simulink model "ROCR6II_URDF_file_915"  (R2020b)
settings: Solver=VariableStepAuto  StartTime=0.0  StopTime=10  FixedStep=0.01  RelTol=1e-3
values from neighbouring files (symbols this model uses):
  X = [x,y,z,Roll,Pitch,Yaw]    [T2RPY.m]
undefined symbols (not defined in the file or in its folder): A, Y, Z
libraries: fl_lib x115, sm_lib x74, nesl_utility x59, fl_ps_legacy_lib x48, ee_lib x12, simulink_extras x7, simulink x6
(part 4 of 5)

== system ROCR6II_URDF_file_915/Driver1/Joint_Driver_5/Controller/Speed/Step Rate and Direction ==
  note: The speed controller turns the reference input into an absolute voltage demand for the
      | voltage-controlled pulse generator and sets the reverse flag signal to +5 volts when the
      | speed demand is negative.
  Reference : Inport
  Abs : Abs
  Compare To Constant : simulink/Logic and Bit Operations/Compare To Constant  relop=<  const=0  OutDataTypeStr=uint8  ZeroCross=off
  Data Type Conversion : DataTypeConversion
  IC Analog Output REV : Subsystem
  IC Analog Output Vref : Subsystem
  Logic2Volts : Gain  Gain=5
  Max step rate 100/s : Saturate  UpperLimit=100  LowerLimit=0
  StepRate2Volts : Gain  Gain=5/100
  REV : PMIOPort  Side=Right
  Vref : PMIOPort  Port=2  Side=Right
  wires:
  Logic2Volts/1 -> IC Analog Output REV/1(SL)
  Abs/1 -> Max step rate 100/s/1
  Reference/1 -> Abs/1, Compare To Constant/1
  Compare To Constant/1 -> Data Type Conversion/1
  Data Type Conversion/1 -> Logic2Volts/1
  Max step rate 100/s/1 -> StepRate2Volts/1
  StepRate2Volts/1 -> IC Analog Output Vref/1(SL)
  connections:
  Vref/RConn1 -- IC Analog Output Vref/RConn1
  REV/RConn1 -- IC Analog Output REV/RConn1

== system ROCR6II_URDF_file_915/Driver1/Joint_Driver_5/Controller/Speed/Voltage-Controlled Pulse Generator ==
  2*pi : fl_ps_legacy_lib/Legacy Physical Signals/Functions/PS Gain  gain=-2*pi
      settings: SourceProductName=Foundation Library
  Controlled Voltage Source : fl_lib/Electrical/Electrical Sources/Controlled Voltage Source
      settings: SourceProductName=Foundation Library
  ERef : fl_lib/Electrical/Electrical Elements/Electrical Reference
      settings: SourceProductName=Foundation Library
  Max step rate =100 : fl_ps_legacy_lib/Legacy Physical Signals/Functions/PS Gain  gain=100
      settings: SourceProductName=Foundation Library
  Normalize to 1 : fl_ps_legacy_lib/Legacy Physical Signals/Functions/PS Gain  gain=1/5
      settings: SourceProductName=Foundation Library
  PS Integrator : fl_ps_legacy_lib/Legacy Physical Signals/Linear Operators/PS Integrator  x0=0
      settings: SourceProductName=Foundation Library  InternalSimscapePortConfiguration="{\"Bottom\":[],\"Left\":[{\"id\":\"I\",\"label\":\"\",\"type\":\"input\"}],\"Right\":[{\"id\":\"O\",\"label\":\"\",\"type\":\"output\"}],\"Top\":[]}"
  PS Sign : fl_ps_legacy_lib/Legacy Physical Signals/Nonlinear Operators/PS Sign
      settings: SourceProductName=Foundation Library  InternalSimscapePortConfiguration="{\"Bottom\":[],\"Left\":[{\"id\":\"I\",\"label\":\"\",\"type\":\"input\"}],\"Right\":[{\"id\":\"O\",\"label\":\"\",\"type\":\"output\"}],\"Top\":[]}"
  PS Sine : fl_ps_legacy_lib/Legacy Physical Signals/Functions/PS Math Function  fcn_choice=1
      settings: SourceProductName=Foundation Library  InternalSimscapePortConfiguration="{\"Bottom\":[],\"Left\":[{\"id\":\"I\",\"label\":\"\",\"type\":\"input\"}],\"Right\":[{\"id\":\"O\",\"label\":\"\",\"type\":\"output\"}],\"Top\":[]}"
  Voltage Sensor : fl_lib/Electrical/Electrical Sensors/Voltage Sensor
      settings: SourceProductName=Foundation Library
  "[0,1]" : fl_ps_legacy_lib/Legacy Physical Signals/Nonlinear Operators/PS Saturation  upper_limit=1  lower_limit=0
      settings: SourceProductName=Foundation Library  InternalSimscapePortConfiguration="{\"Bottom\":[],\"Left\":[{\"id\":\"I\",\"label\":\"\",\"type\":\"input\"}],\"Right\":[{\"id\":\"O\",\"label\":\"\",\"type\":\"output\"}],\"Top\":[]}"
  logic2volts : fl_ps_legacy_lib/Legacy Physical Signals/Functions/PS Gain  gain=5
      settings: SourceProductName=Foundation Library
  PWM : PMIOPort  Side=Right
  0v : PMIOPort  Port=2  Side=Right
  Vref : PMIOPort  Port=3  Side=Left
  connections:
  logic2volts/RConn1 -- Controlled Voltage Source/RConn1
  "[0,1]"/RConn1 -- logic2volts/LConn1
  "[0,1]"/LConn1 -- PS Sign/RConn1
  PS Sign/LConn1 -- PS Sine/RConn1
  PS Integrator/RConn1 -- PS Sine/LConn1
  2*pi/RConn1 -- PS Integrator/LConn1
  Max step rate =100/RConn1 -- 2*pi/LConn1
  Max step rate =100/LConn1 -- Normalize to 1/RConn1
  Voltage Sensor/RConn1 -- Normalize to 1/LConn1
  ERef/LConn1 -- Voltage Sensor/RConn2
  Vref/RConn1 -- Voltage Sensor/LConn1
  Controlled Voltage Source/RConn2 -- 0v/RConn1
  PWM/RConn1 -- Controlled Voltage Source/LConn1

== system ROCR6II_URDF_file_915/Driver1/Joint_Driver_6/Controller/Position/Algorithm and Pulse Generation ==
  note: The reference input defines the required angular position in terms of
      | the number steps. For this stepper, the step size is 1.8 degrees. Hence
      | a demand of 10 steps results in an angle change of 18 degrees.
      | The step rate is set by the Pulse Generator's Pulse rate mask parameter.
  note: Position Controller
  Reference : Inport
  IC Analog Output REV : Subsystem
  IC Analog Output Vref : Subsystem
  Logic2Volts1 : Gain  Gain=5
  Logic2Volts2 : Gain  Gain=5
  Pulse Generator : Subsystem  mask{f=20}
      mask prompts: f "Pulse rate"
  Rate Transition : RateTransition  Deterministic=off
  REV : PMIOPort  Side=Right
  Vref : PMIOPort  Port=2  Side=Right
  wires:
  Logic2Volts1/1 -> IC Analog Output Vref/1(SL)
  Pulse Generator/1(Pulse train) -> Logic2Volts1/1
  Reference/1 -> Rate Transition/1
  Logic2Volts2/1 -> IC Analog Output REV/1(SL)
  Pulse Generator/2(Pulse direction) -> Logic2Volts2/1
  Rate Transition/1 -> Pulse Generator/1(Pulse  demand)
  connections:
  Vref/RConn1 -- IC Analog Output Vref/RConn1
  REV/RConn1 -- IC Analog Output REV/RConn1

== system ROCR6II_URDF_file_915/Driver1/Joint_Driver_6/Controller/Speed/Step Rate and Direction ==
  note: The speed controller turns the reference input into an absolute voltage demand for the
      | voltage-controlled pulse generator and sets the reverse flag signal to +5 volts when the
      | speed demand is negative.
  Reference : Inport
  Abs : Abs
  Compare To Constant : simulink/Logic and Bit Operations/Compare To Constant  relop=<  const=0  OutDataTypeStr=uint8  ZeroCross=off
  Data Type Conversion : DataTypeConversion
  IC Analog Output REV : Subsystem
  IC Analog Output Vref : Subsystem
  Logic2Volts : Gain  Gain=5
  Max step rate 100/s : Saturate  UpperLimit=100  LowerLimit=0
  StepRate2Volts : Gain  Gain=5/100
  REV : PMIOPort  Side=Right
  Vref : PMIOPort  Port=2  Side=Right
  wires:
  StepRate2Volts/1 -> IC Analog Output Vref/1(SL)
  Max step rate 100/s/1 -> StepRate2Volts/1
  Data Type Conversion/1 -> Logic2Volts/1
  Compare To Constant/1 -> Data Type Conversion/1
  Reference/1 -> Compare To Constant/1, Abs/1
  Abs/1 -> Max step rate 100/s/1
  Logic2Volts/1 -> IC Analog Output REV/1(SL)
  connections:
  REV/RConn1 -- IC Analog Output REV/RConn1
  Vref/RConn1 -- IC Analog Output Vref/RConn1

== system ROCR6II_URDF_file_915/Driver1/Joint_Driver_6/Controller/Speed/Voltage-Controlled Pulse Generator ==
  2*pi : fl_ps_legacy_lib/Legacy Physical Signals/Functions/PS Gain  gain=-2*pi
      settings: SourceProductName=Foundation Library
  Controlled Voltage Source : fl_lib/Electrical/Electrical Sources/Controlled Voltage Source
      settings: SourceProductName=Foundation Library
  ERef : fl_lib/Electrical/Electrical Elements/Electrical Reference
      settings: SourceProductName=Foundation Library
  Max step rate =100 : fl_ps_legacy_lib/Legacy Physical Signals/Functions/PS Gain  gain=100
      settings: SourceProductName=Foundation Library
  Normalize to 1 : fl_ps_legacy_lib/Legacy Physical Signals/Functions/PS Gain  gain=1/5
      settings: SourceProductName=Foundation Library
  PS Integrator : fl_ps_legacy_lib/Legacy Physical Signals/Linear Operators/PS Integrator  x0=0
      settings: SourceProductName=Foundation Library  InternalSimscapePortConfiguration="{\"Bottom\":[],\"Left\":[{\"id\":\"I\",\"label\":\"\",\"type\":\"input\"}],\"Right\":[{\"id\":\"O\",\"label\":\"\",\"type\":\"output\"}],\"Top\":[]}"
  PS Sign : fl_ps_legacy_lib/Legacy Physical Signals/Nonlinear Operators/PS Sign
      settings: SourceProductName=Foundation Library  InternalSimscapePortConfiguration="{\"Bottom\":[],\"Left\":[{\"id\":\"I\",\"label\":\"\",\"type\":\"input\"}],\"Right\":[{\"id\":\"O\",\"label\":\"\",\"type\":\"output\"}],\"Top\":[]}"
  PS Sine : fl_ps_legacy_lib/Legacy Physical Signals/Functions/PS Math Function  fcn_choice=1
      settings: SourceProductName=Foundation Library  InternalSimscapePortConfiguration="{\"Bottom\":[],\"Left\":[{\"id\":\"I\",\"label\":\"\",\"type\":\"input\"}],\"Right\":[{\"id\":\"O\",\"label\":\"\",\"type\":\"output\"}],\"Top\":[]}"
  Voltage Sensor : fl_lib/Electrical/Electrical Sensors/Voltage Sensor
      settings: SourceProductName=Foundation Library
  "[0,1]" : fl_ps_legacy_lib/Legacy Physical Signals/Nonlinear Operators/PS Saturation  upper_limit=1  lower_limit=0
      settings: SourceProductName=Foundation Library  InternalSimscapePortConfiguration="{\"Bottom\":[],\"Left\":[{\"id\":\"I\",\"label\":\"\",\"type\":\"input\"}],\"Right\":[{\"id\":\"O\",\"label\":\"\",\"type\":\"output\"}],\"Top\":[]}"
  logic2volts : fl_ps_legacy_lib/Legacy Physical Signals/Functions/PS Gain  gain=5
      settings: SourceProductName=Foundation Library
  PWM : PMIOPort  Side=Right
  0v : PMIOPort  Port=2  Side=Right
  Vref : PMIOPort  Port=3  Side=Left
  connections:
  PWM/RConn1 -- Controlled Voltage Source/LConn1
  Controlled Voltage Source/RConn2 -- 0v/RConn1
  Vref/RConn1 -- Voltage Sensor/LConn1
  ERef/LConn1 -- Voltage Sensor/RConn2
  Voltage Sensor/RConn1 -- Normalize to 1/LConn1
  Max step rate =100/LConn1 -- Normalize to 1/RConn1
  Max step rate =100/RConn1 -- 2*pi/LConn1
  2*pi/RConn1 -- PS Integrator/LConn1
  PS Integrator/RConn1 -- PS Sine/LConn1
  PS Sign/LConn1 -- PS Sine/RConn1
  "[0,1]"/LConn1 -- PS Sign/RConn1
  "[0,1]"/RConn1 -- logic2volts/LConn1
  logic2volts/RConn1 -- Controlled Voltage Source/RConn1

== system ROCR6II_URDF_file_915/Driver1/Joint_Driver_1/Controller/Position/Algorithm and Pulse Generation/IC Analog Output REV ==
  SL : Inport
  Controlled Voltage Source : fl_lib/Electrical/Electrical Sources/Controlled Voltage Source
      settings: SourceProductName=Foundation Library
  ERef : fl_lib/Electrical/Electrical Elements/Electrical Reference
      settings: SourceProductName=Foundation Library
  Simulink-PS Converter : nesl_utility/Simulink-PS Converter  PhysicalDomain=network_engine_domain  SubClassName=ps_input  LeftPortType=input  RightPortType=output  PseudoPeriodic=off  Frequencies=[]  NoiseDistribution=none  NoiseParameters=[]  Unit=V  AffineConversion=off  FilteringAndDerivatives=zero  SimscapeFilterOrder=1  InputFilterTimeConstant=.001  UdotUserProvided=0
  V : PMIOPort  Side=Right
  wires:
  SL/1 -> Simulink-PS Converter/1
  connections:
  Simulink-PS Converter/RConn1 -- Controlled Voltage Source/RConn1
  V/RConn1 -- Controlled Voltage Source/LConn1
  ERef/LConn1 -- Controlled Voltage Source/RConn2

== system ROCR6II_URDF_file_915/Driver1/Joint_Driver_1/Controller/Position/Algorithm and Pulse Generation/IC Analog Output Vref ==
  SL : Inport
  Controlled Voltage Source : fl_lib/Electrical/Electrical Sources/Controlled Voltage Source
      settings: SourceProductName=Foundation Library
  ERef : fl_lib/Electrical/Electrical Elements/Electrical Reference
      settings: SourceProductName=Foundation Library
  Simulink-PS Converter : nesl_utility/Simulink-PS Converter  PhysicalDomain=network_engine_domain  SubClassName=ps_input  LeftPortType=input  RightPortType=output  PseudoPeriodic=off  Frequencies=[]  NoiseDistribution=none  NoiseParameters=[]  Unit=V  AffineConversion=off  FilteringAndDerivatives=zero  SimscapeFilterOrder=1  InputFilterTimeConstant=.001  UdotUserProvided=0
  V : PMIOPort  Side=Right
  wires:
  SL/1 -> Simulink-PS Converter/1
  connections:
  ERef/LConn1 -- Controlled Voltage Source/RConn2
  V/RConn1 -- Controlled Voltage Source/LConn1
  Simulink-PS Converter/RConn1 -- Controlled Voltage Source/RConn1

== system ROCR6II_URDF_file_915/Driver1/Joint_Driver_1/Controller/Position/Algorithm and Pulse Generation/Pulse Generator ==
  Pulse  demand : Inport  SampleTime=1/f
  -1 : Gain  Gain=-1
  Abs : Abs
  Product : Product  InputSameDT=on  SaturateOnIntegerOverflow=on  OutDataTypeStr=Inherit: Same as first input
  Pulse Generator : Subsystem
  Rate Transition : RateTransition  Deterministic=off
  Saturation : Saturate  UpperLimit=1  LowerLimit=-1
  Sign : Signum
  Sum : Sum  Inputs=|+-
  Sum1 : Sum  Inputs=|++
  "Unit Delay, sample time 1/f" : UnitDelay  SampleTime=1/f  HasFrameUpgradeWarning=on
  "[0,1]" : Saturate  UpperLimit=1  LowerLimit=0
  Pulse train : Outport  VectorParamsAs1DForOutWhenUnconnected=off
  Pulse direction : Outport  Port=2  VectorParamsAs1DForOutWhenUnconnected=off
  wires:
  Rate Transition/1 -> Product/1
  Pulse Generator/1(p) -> Product/2
  Abs/1 -> Rate Transition/1
  Product/1 -> Pulse train/1
  Sign/1 -> "[0,1]"/1
  Sum1/1 -> "Unit Delay, sample time 1/f"/1
  Saturation/1 -> Abs/1, Sum1/1
  Sum/1 -> Saturation/1, -1/1
  Pulse  demand/1 -> Sum/1
  "Unit Delay, sample time 1/f"/1 -> Sum1/2, Sum/2
  -1/1 -> Sign/1
  "[0,1]"/1 -> Pulse direction/1

== system ROCR6II_URDF_file_915/Driver1/Joint_Driver_1/Controller/Speed/Step Rate and Direction/IC Analog Output REV ==
  SL : Inport
  Controlled Voltage Source : fl_lib/Electrical/Electrical Sources/Controlled Voltage Source
      settings: SourceProductName=Foundation Library
  ERef : fl_lib/Electrical/Electrical Elements/Electrical Reference
      settings: SourceProductName=Foundation Library
  Simulink-PS Converter : nesl_utility/Simulink-PS Converter  PhysicalDomain=network_engine_domain  SubClassName=ps_input  LeftPortType=input  RightPortType=output  PseudoPeriodic=off  Frequencies=[]  NoiseDistribution=none  NoiseParameters=[]  Unit=V  AffineConversion=off  FilteringAndDerivatives=zero  SimscapeFilterOrder=1  InputFilterTimeConstant=.001  UdotUserProvided=0
  V : PMIOPort  Side=Right
  wires:
  SL/1 -> Simulink-PS Converter/1
  connections:
  ERef/LConn1 -- Controlled Voltage Source/RConn2
  V/RConn1 -- Controlled Voltage Source/LConn1
  Simulink-PS Converter/RConn1 -- Controlled Voltage Source/RConn1

== system ROCR6II_URDF_file_915/Driver1/Joint_Driver_1/Controller/Speed/Step Rate and Direction/IC Analog Output Vref ==
  SL : Inport
  Controlled Voltage Source : fl_lib/Electrical/Electrical Sources/Controlled Voltage Source
      settings: SourceProductName=Foundation Library
  ERef : fl_lib/Electrical/Electrical Elements/Electrical Reference
      settings: SourceProductName=Foundation Library
  Simulink-PS Converter : nesl_utility/Simulink-PS Converter  PhysicalDomain=network_engine_domain  SubClassName=ps_input  LeftPortType=input  RightPortType=output  PseudoPeriodic=off  Frequencies=[]  NoiseDistribution=none  NoiseParameters=[]  Unit=V  AffineConversion=off  FilteringAndDerivatives=zero  SimscapeFilterOrder=1  InputFilterTimeConstant=.001  UdotUserProvided=0
  V : PMIOPort  Side=Right
  wires:
  SL/1 -> Simulink-PS Converter/1
  connections:
  Simulink-PS Converter/RConn1 -- Controlled Voltage Source/RConn1
  V/RConn1 -- Controlled Voltage Source/LConn1
  ERef/LConn1 -- Controlled Voltage Source/RConn2

== system ROCR6II_URDF_file_915/Driver1/Joint_Driver_2/Controller/Position/Algorithm and Pulse Generation/IC Analog Output REV ==
  SL : Inport
  Controlled Voltage Source : fl_lib/Electrical/Electrical Sources/Controlled Voltage Source
      settings: SourceProductName=Foundation Library
  ERef : fl_lib/Electrical/Electrical Elements/Electrical Reference
      settings: SourceProductName=Foundation Library
  Simulink-PS Converter : nesl_utility/Simulink-PS Converter  PhysicalDomain=network_engine_domain  SubClassName=ps_input  LeftPortType=input  RightPortType=output  PseudoPeriodic=off  Frequencies=[]  NoiseDistribution=none  NoiseParameters=[]  Unit=V  AffineConversion=off  FilteringAndDerivatives=zero  SimscapeFilterOrder=1  InputFilterTimeConstant=.001  UdotUserProvided=0
  V : PMIOPort  Side=Right
  wires:
  SL/1 -> Simulink-PS Converter/1
  connections:
  ERef/LConn1 -- Controlled Voltage Source/RConn2
  V/RConn1 -- Controlled Voltage Source/LConn1
  Simulink-PS Converter/RConn1 -- Controlled Voltage Source/RConn1

== system ROCR6II_URDF_file_915/Driver1/Joint_Driver_2/Controller/Position/Algorithm and Pulse Generation/IC Analog Output Vref ==
  SL : Inport
  Controlled Voltage Source : fl_lib/Electrical/Electrical Sources/Controlled Voltage Source
      settings: SourceProductName=Foundation Library
  ERef : fl_lib/Electrical/Electrical Elements/Electrical Reference
      settings: SourceProductName=Foundation Library
  Simulink-PS Converter : nesl_utility/Simulink-PS Converter  PhysicalDomain=network_engine_domain  SubClassName=ps_input  LeftPortType=input  RightPortType=output  PseudoPeriodic=off  Frequencies=[]  NoiseDistribution=none  NoiseParameters=[]  Unit=V  AffineConversion=off  FilteringAndDerivatives=zero  SimscapeFilterOrder=1  InputFilterTimeConstant=.001  UdotUserProvided=0
  V : PMIOPort  Side=Right
  wires:
  SL/1 -> Simulink-PS Converter/1
  connections:
  Simulink-PS Converter/RConn1 -- Controlled Voltage Source/RConn1
  V/RConn1 -- Controlled Voltage Source/LConn1
  ERef/LConn1 -- Controlled Voltage Source/RConn2

== system ROCR6II_URDF_file_915/Driver1/Joint_Driver_2/Controller/Position/Algorithm and Pulse Generation/Pulse Generator ==
  Pulse  demand : Inport  SampleTime=1/f
  -1 : Gain  Gain=-1
  Abs : Abs
  Product : Product  InputSameDT=on  SaturateOnIntegerOverflow=on  OutDataTypeStr=Inherit: Same as first input
  Pulse Generator : Subsystem
  Rate Transition : RateTransition  Deterministic=off
  Saturation : Saturate  UpperLimit=1  LowerLimit=-1
  Sign : Signum
  Sum : Sum  Inputs=|+-
  Sum1 : Sum  Inputs=|++
  "Unit Delay, sample time 1/f" : UnitDelay  SampleTime=1/f  HasFrameUpgradeWarning=on
  "[0,1]" : Saturate  UpperLimit=1  LowerLimit=0
  Pulse train : Outport  VectorParamsAs1DForOutWhenUnconnected=off
  Pulse direction : Outport  Port=2  VectorParamsAs1DForOutWhenUnconnected=off
  wires:
  "[0,1]"/1 -> Pulse direction/1
  -1/1 -> Sign/1
  "Unit Delay, sample time 1/f"/1 -> Sum/2, Sum1/2
  Pulse  demand/1 -> Sum/1
  Sum/1 -> -1/1, Saturation/1
  Saturation/1 -> Sum1/1, Abs/1
  Sum1/1 -> "Unit Delay, sample time 1/f"/1
  Sign/1 -> "[0,1]"/1
  Product/1 -> Pulse train/1
  Abs/1 -> Rate Transition/1
  Pulse Generator/1(p) -> Product/2
  Rate Transition/1 -> Product/1

== system ROCR6II_URDF_file_915/Driver1/Joint_Driver_2/Controller/Speed/Step Rate and Direction/IC Analog Output REV ==
  SL : Inport
  Controlled Voltage Source : fl_lib/Electrical/Electrical Sources/Controlled Voltage Source
      settings: SourceProductName=Foundation Library
  ERef : fl_lib/Electrical/Electrical Elements/Electrical Reference
      settings: SourceProductName=Foundation Library
  Simulink-PS Converter : nesl_utility/Simulink-PS Converter  PhysicalDomain=network_engine_domain  SubClassName=ps_input  LeftPortType=input  RightPortType=output  PseudoPeriodic=off  Frequencies=[]  NoiseDistribution=none  NoiseParameters=[]  Unit=V  AffineConversion=off  FilteringAndDerivatives=zero  SimscapeFilterOrder=1  InputFilterTimeConstant=.001  UdotUserProvided=0
  V : PMIOPort  Side=Right
  wires:
  SL/1 -> Simulink-PS Converter/1
  connections:
  Simulink-PS Converter/RConn1 -- Controlled Voltage Source/RConn1
  V/RConn1 -- Controlled Voltage Source/LConn1
  ERef/LConn1 -- Controlled Voltage Source/RConn2

== system ROCR6II_URDF_file_915/Driver1/Joint_Driver_2/Controller/Speed/Step Rate and Direction/IC Analog Output Vref ==
  SL : Inport
  Controlled Voltage Source : fl_lib/Electrical/Electrical Sources/Controlled Voltage Source
      settings: SourceProductName=Foundation Library
  ERef : fl_lib/Electrical/Electrical Elements/Electrical Reference
      settings: SourceProductName=Foundation Library
  Simulink-PS Converter : nesl_utility/Simulink-PS Converter  PhysicalDomain=network_engine_domain  SubClassName=ps_input  LeftPortType=input  RightPortType=output  PseudoPeriodic=off  Frequencies=[]  NoiseDistribution=none  NoiseParameters=[]  Unit=V  AffineConversion=off  FilteringAndDerivatives=zero  SimscapeFilterOrder=1  InputFilterTimeConstant=.001  UdotUserProvided=0
  V : PMIOPort  Side=Right
  wires:
  SL/1 -> Simulink-PS Converter/1
  connections:
  ERef/LConn1 -- Controlled Voltage Source/RConn2
  V/RConn1 -- Controlled Voltage Source/LConn1
  Simulink-PS Converter/RConn1 -- Controlled Voltage Source/RConn1

== system ROCR6II_URDF_file_915/Driver1/Joint_Driver_3/Controller/Position/Algorithm and Pulse Generation/IC Analog Output REV ==
  SL : Inport
  Controlled Voltage Source : fl_lib/Electrical/Electrical Sources/Controlled Voltage Source
      settings: SourceProductName=Foundation Library
  ERef : fl_lib/Electrical/Electrical Elements/Electrical Reference
      settings: SourceProductName=Foundation Library
  Simulink-PS Converter : nesl_utility/Simulink-PS Converter  PhysicalDomain=network_engine_domain  SubClassName=ps_input  LeftPortType=input  RightPortType=output  PseudoPeriodic=off  Frequencies=[]  NoiseDistribution=none  NoiseParameters=[]  Unit=V  AffineConversion=off  FilteringAndDerivatives=zero  SimscapeFilterOrder=1  InputFilterTimeConstant=.001  UdotUserProvided=0
  V : PMIOPort  Side=Right
  wires:
  SL/1 -> Simulink-PS Converter/1
  connections:
  Simulink-PS Converter/RConn1 -- Controlled Voltage Source/RConn1
  V/RConn1 -- Controlled Voltage Source/LConn1
  ERef/LConn1 -- Controlled Voltage Source/RConn2

== system ROCR6II_URDF_file_915/Driver1/Joint_Driver_3/Controller/Position/Algorithm and Pulse Generation/IC Analog Output Vref ==
  SL : Inport
  Controlled Voltage Source : fl_lib/Electrical/Electrical Sources/Controlled Voltage Source
      settings: SourceProductName=Foundation Library
  ERef : fl_lib/Electrical/Electrical Elements/Electrical Reference
      settings: SourceProductName=Foundation Library
  Simulink-PS Converter : nesl_utility/Simulink-PS Converter  PhysicalDomain=network_engine_domain  SubClassName=ps_input  LeftPortType=input  RightPortType=output  PseudoPeriodic=off  Frequencies=[]  NoiseDistribution=none  NoiseParameters=[]  Unit=V  AffineConversion=off  FilteringAndDerivatives=zero  SimscapeFilterOrder=1  InputFilterTimeConstant=.001  UdotUserProvided=0
  V : PMIOPort  Side=Right
  wires:
  SL/1 -> Simulink-PS Converter/1
  connections:
  ERef/LConn1 -- Controlled Voltage Source/RConn2
  V/RConn1 -- Controlled Voltage Source/LConn1
  Simulink-PS Converter/RConn1 -- Controlled Voltage Source/RConn1

== system ROCR6II_URDF_file_915/Driver1/Joint_Driver_3/Controller/Position/Algorithm and Pulse Generation/Pulse Generator ==
  Pulse  demand : Inport  SampleTime=1/f
  -1 : Gain  Gain=-1
  Abs : Abs
  Product : Product  InputSameDT=on  SaturateOnIntegerOverflow=on  OutDataTypeStr=Inherit: Same as first input
  Pulse Generator : Subsystem
  Rate Transition : RateTransition  Deterministic=off
  Saturation : Saturate  UpperLimit=1  LowerLimit=-1
  Sign : Signum
  Sum : Sum  Inputs=|+-
  Sum1 : Sum  Inputs=|++
  "Unit Delay, sample time 1/f" : UnitDelay  SampleTime=1/f  HasFrameUpgradeWarning=on
  "[0,1]" : Saturate  UpperLimit=1  LowerLimit=0
  Pulse train : Outport  VectorParamsAs1DForOutWhenUnconnected=off
  Pulse direction : Outport  Port=2  VectorParamsAs1DForOutWhenUnconnected=off
  wires:
  Rate Transition/1 -> Product/1
  Pulse Generator/1(p) -> Product/2
  Abs/1 -> Rate Transition/1
  Product/1 -> Pulse train/1
  Sign/1 -> "[0,1]"/1
  Sum1/1 -> "Unit Delay, sample time 1/f"/1
  Saturation/1 -> Abs/1, Sum1/1
  Sum/1 -> Saturation/1, -1/1
  Pulse  demand/1 -> Sum/1
  "Unit Delay, sample time 1/f"/1 -> Sum1/2, Sum/2
  -1/1 -> Sign/1
  "[0,1]"/1 -> Pulse direction/1

== system ROCR6II_URDF_file_915/Driver1/Joint_Driver_3/Controller/Speed/Step Rate and Direction/IC Analog Output REV ==
  SL : Inport
  Controlled Voltage Source : fl_lib/Electrical/Electrical Sources/Controlled Voltage Source
      settings: SourceProductName=Foundation Library
  ERef : fl_lib/Electrical/Electrical Elements/Electrical Reference
      settings: SourceProductName=Foundation Library
  Simulink-PS Converter : nesl_utility/Simulink-PS Converter  PhysicalDomain=network_engine_domain  SubClassName=ps_input  LeftPortType=input  RightPortType=output  PseudoPeriodic=off  Frequencies=[]  NoiseDistribution=none  NoiseParameters=[]  Unit=V  AffineConversion=off  FilteringAndDerivatives=zero  SimscapeFilterOrder=1  InputFilterTimeConstant=.001  UdotUserProvided=0
  V : PMIOPort  Side=Right
  wires:
  SL/1 -> Simulink-PS Converter/1
  connections:
  ERef/LConn1 -- Controlled Voltage Source/RConn2
  V/RConn1 -- Controlled Voltage Source/LConn1
  Simulink-PS Converter/RConn1 -- Controlled Voltage Source/RConn1

== system ROCR6II_URDF_file_915/Driver1/Joint_Driver_3/Controller/Speed/Step Rate and Direction/IC Analog Output Vref ==
  SL : Inport
  Controlled Voltage Source : fl_lib/Electrical/Electrical Sources/Controlled Voltage Source
      settings: SourceProductName=Foundation Library
  ERef : fl_lib/Electrical/Electrical Elements/Electrical Reference
      settings: SourceProductName=Foundation Library
  Simulink-PS Converter : nesl_utility/Simulink-PS Converter  PhysicalDomain=network_engine_domain  SubClassName=ps_input  LeftPortType=input  RightPortType=output  PseudoPeriodic=off  Frequencies=[]  NoiseDistribution=none  NoiseParameters=[]  Unit=V  AffineConversion=off  FilteringAndDerivatives=zero  SimscapeFilterOrder=1  InputFilterTimeConstant=.001  UdotUserProvided=0
  V : PMIOPort  Side=Right
  wires:
  SL/1 -> Simulink-PS Converter/1
  connections:
  Simulink-PS Converter/RConn1 -- Controlled Voltage Source/RConn1
  V/RConn1 -- Controlled Voltage Source/LConn1
  ERef/LConn1 -- Controlled Voltage Source/RConn2

== system ROCR6II_URDF_file_915/Driver1/Joint_Driver_4/Controller/Position/Algorithm and Pulse Generation/IC Analog Output REV ==
  SL : Inport
  Controlled Voltage Source : fl_lib/Electrical/Electrical Sources/Controlled Voltage Source
      settings: SourceProductName=Foundation Library
  ERef : fl_lib/Electrical/Electrical Elements/Electrical Reference
      settings: SourceProductName=Foundation Library
  Simulink-PS Converter : nesl_utility/Simulink-PS Converter  PhysicalDomain=network_engine_domain  SubClassName=ps_input  LeftPortType=input  RightPortType=output  PseudoPeriodic=off  Frequencies=[]  NoiseDistribution=none  NoiseParameters=[]  Unit=V  AffineConversion=off  FilteringAndDerivatives=zero  SimscapeFilterOrder=1  InputFilterTimeConstant=.001  UdotUserProvided=0
  V : PMIOPort  Side=Right
  wires:
  SL/1 -> Simulink-PS Converter/1
  connections:
  ERef/LConn1 -- Controlled Voltage Source/RConn2
  V/RConn1 -- Controlled Voltage Source/LConn1
  Simulink-PS Converter/RConn1 -- Controlled Voltage Source/RConn1

== system ROCR6II_URDF_file_915/Driver1/Joint_Driver_4/Controller/Position/Algorithm and Pulse Generation/IC Analog Output Vref ==
  SL : Inport
  Controlled Voltage Source : fl_lib/Electrical/Electrical Sources/Controlled Voltage Source
      settings: SourceProductName=Foundation Library
  ERef : fl_lib/Electrical/Electrical Elements/Electrical Reference
      settings: SourceProductName=Foundation Library
  Simulink-PS Converter : nesl_utility/Simulink-PS Converter  PhysicalDomain=network_engine_domain  SubClassName=ps_input  LeftPortType=input  RightPortType=output  PseudoPeriodic=off  Frequencies=[]  NoiseDistribution=none  NoiseParameters=[]  Unit=V  AffineConversion=off  FilteringAndDerivatives=zero  SimscapeFilterOrder=1  InputFilterTimeConstant=.001  UdotUserProvided=0
  V : PMIOPort  Side=Right
  wires:
  SL/1 -> Simulink-PS Converter/1
  connections:
  Simulink-PS Converter/RConn1 -- Controlled Voltage Source/RConn1
  V/RConn1 -- Controlled Voltage Source/LConn1
  ERef/LConn1 -- Controlled Voltage Source/RConn2

== system ROCR6II_URDF_file_915/Driver1/Joint_Driver_4/Controller/Position/Algorithm and Pulse Generation/Pulse Generator ==
  Pulse  demand : Inport  SampleTime=1/f
  -1 : Gain  Gain=-1
  Abs : Abs
  Product : Product  InputSameDT=on  SaturateOnIntegerOverflow=on  OutDataTypeStr=Inherit: Same as first input
  Pulse Generator : Subsystem
  Rate Transition : RateTransition  Deterministic=off
  Saturation : Saturate  UpperLimit=1  LowerLimit=-1
  Sign : Signum
  Sum : Sum  Inputs=|+-
  Sum1 : Sum  Inputs=|++
  "Unit Delay, sample time 1/f" : UnitDelay  SampleTime=1/f  HasFrameUpgradeWarning=on
  "[0,1]" : Saturate  UpperLimit=1  LowerLimit=0
  Pulse train : Outport  VectorParamsAs1DForOutWhenUnconnected=off
  Pulse direction : Outport  Port=2  VectorParamsAs1DForOutWhenUnconnected=off
  wires:
  "[0,1]"/1 -> Pulse direction/1
  -1/1 -> Sign/1
  "Unit Delay, sample time 1/f"/1 -> Sum/2, Sum1/2
  Pulse  demand/1 -> Sum/1
  Sum/1 -> -1/1, Saturation/1
  Saturation/1 -> Sum1/1, Abs/1
  Sum1/1 -> "Unit Delay, sample time 1/f"/1
  Sign/1 -> "[0,1]"/1
  Product/1 -> Pulse train/1
  Abs/1 -> Rate Transition/1
  Pulse Generator/1(p) -> Product/2
  Rate Transition/1 -> Product/1

== system ROCR6II_URDF_file_915/Driver1/Joint_Driver_4/Controller/Speed/Step Rate and Direction/IC Analog Output REV ==
  SL : Inport
  Controlled Voltage Source : fl_lib/Electrical/Electrical Sources/Controlled Voltage Source
      settings: SourceProductName=Foundation Library
  ERef : fl_lib/Electrical/Electrical Elements/Electrical Reference
      settings: SourceProductName=Foundation Library
  Simulink-PS Converter : nesl_utility/Simulink-PS Converter  PhysicalDomain=network_engine_domain  SubClassName=ps_input  LeftPortType=input  RightPortType=output  PseudoPeriodic=off  Frequencies=[]  NoiseDistribution=none  NoiseParameters=[]  Unit=V  AffineConversion=off  FilteringAndDerivatives=zero  SimscapeFilterOrder=1  InputFilterTimeConstant=.001  UdotUserProvided=0
  V : PMIOPort  Side=Right
  wires:
  SL/1 -> Simulink-PS Converter/1
  connections:
  Simulink-PS Converter/RConn1 -- Controlled Voltage Source/RConn1
  V/RConn1 -- Controlled Voltage Source/LConn1
  ERef/LConn1 -- Controlled Voltage Source/RConn2

== system ROCR6II_URDF_file_915/Driver1/Joint_Driver_4/Controller/Speed/Step Rate and Direction/IC Analog Output Vref ==
  SL : Inport
  Controlled Voltage Source : fl_lib/Electrical/Electrical Sources/Controlled Voltage Source
      settings: SourceProductName=Foundation Library
  ERef : fl_lib/Electrical/Electrical Elements/Electrical Reference
      settings: SourceProductName=Foundation Library
  Simulink-PS Converter : nesl_utility/Simulink-PS Converter  PhysicalDomain=network_engine_domain  SubClassName=ps_input  LeftPortType=input  RightPortType=output  PseudoPeriodic=off  Frequencies=[]  NoiseDistribution=none  NoiseParameters=[]  Unit=V  AffineConversion=off  FilteringAndDerivatives=zero  SimscapeFilterOrder=1  InputFilterTimeConstant=.001  UdotUserProvided=0
  V : PMIOPort  Side=Right
  wires:
  SL/1 -> Simulink-PS Converter/1
  connections:
  ERef/LConn1 -- Controlled Voltage Source/RConn2
  V/RConn1 -- Controlled Voltage Source/LConn1
  Simulink-PS Converter/RConn1 -- Controlled Voltage Source/RConn1

== system ROCR6II_URDF_file_915/Driver1/Joint_Driver_5/Controller/Position/Algorithm and Pulse Generation/IC Analog Output REV ==
  SL : Inport
  Controlled Voltage Source : fl_lib/Electrical/Electrical Sources/Controlled Voltage Source
      settings: SourceProductName=Foundation Library
  ERef : fl_lib/Electrical/Electrical Elements/Electrical Reference
      settings: SourceProductName=Foundation Library
  Simulink-PS Converter : nesl_utility/Simulink-PS Converter  PhysicalDomain=network_engine_domain  SubClassName=ps_input  LeftPortType=input  RightPortType=output  PseudoPeriodic=off  Frequencies=[]  NoiseDistribution=none  NoiseParameters=[]  Unit=V  AffineConversion=off  FilteringAndDerivatives=zero  SimscapeFilterOrder=1  InputFilterTimeConstant=.001  UdotUserProvided=0
  V : PMIOPort  Side=Right
  wires:
  SL/1 -> Simulink-PS Converter/1
  connections:
  Simulink-PS Converter/RConn1 -- Controlled Voltage Source/RConn1
  V/RConn1 -- Controlled Voltage Source/LConn1
  ERef/LConn1 -- Controlled Voltage Source/RConn2

== system ROCR6II_URDF_file_915/Driver1/Joint_Driver_5/Controller/Position/Algorithm and Pulse Generation/IC Analog Output Vref ==
  SL : Inport
  Controlled Voltage Source : fl_lib/Electrical/Electrical Sources/Controlled Voltage Source
      settings: SourceProductName=Foundation Library
  ERef : fl_lib/Electrical/Electrical Elements/Electrical Reference
      settings: SourceProductName=Foundation Library
  Simulink-PS Converter : nesl_utility/Simulink-PS Converter  PhysicalDomain=network_engine_domain  SubClassName=ps_input  LeftPortType=input  RightPortType=output  PseudoPeriodic=off  Frequencies=[]  NoiseDistribution=none  NoiseParameters=[]  Unit=V  AffineConversion=off  FilteringAndDerivatives=zero  SimscapeFilterOrder=1  InputFilterTimeConstant=.001  UdotUserProvided=0
  V : PMIOPort  Side=Right
  wires:
  SL/1 -> Simulink-PS Converter/1
  connections:
  ERef/LConn1 -- Controlled Voltage Source/RConn2
  V/RConn1 -- Controlled Voltage Source/LConn1
  Simulink-PS Converter/RConn1 -- Controlled Voltage Source/RConn1

== system ROCR6II_URDF_file_915/Driver1/Joint_Driver_5/Controller/Position/Algorithm and Pulse Generation/Pulse Generator ==
  Pulse  demand : Inport  SampleTime=1/f
  -1 : Gain  Gain=-1
  Abs : Abs
  Product : Product  InputSameDT=on  SaturateOnIntegerOverflow=on  OutDataTypeStr=Inherit: Same as first input
  Pulse Generator : Subsystem
  Rate Transition : RateTransition  Deterministic=off
  Saturation : Saturate  UpperLimit=1  LowerLimit=-1
  Sign : Signum
  Sum : Sum  Inputs=|+-
  Sum1 : Sum  Inputs=|++
  "Unit Delay, sample time 1/f" : UnitDelay  SampleTime=1/f  HasFrameUpgradeWarning=on
  "[0,1]" : Saturate  UpperLimit=1  LowerLimit=0
  Pulse train : Outport  VectorParamsAs1DForOutWhenUnconnected=off
  Pulse direction : Outport  Port=2  VectorParamsAs1DForOutWhenUnconnected=off
  wires:
  Rate Transition/1 -> Product/1
  Pulse Generator/1(p) -> Product/2
  Abs/1 -> Rate Transition/1
  Product/1 -> Pulse train/1
  Sign/1 -> "[0,1]"/1
  Sum1/1 -> "Unit Delay, sample time 1/f"/1
  Saturation/1 -> Abs/1, Sum1/1
  Sum/1 -> Saturation/1, -1/1
  Pulse  demand/1 -> Sum/1
  "Unit Delay, sample time 1/f"/1 -> Sum1/2, Sum/2
  -1/1 -> Sign/1
  "[0,1]"/1 -> Pulse direction/1

== system ROCR6II_URDF_file_915/Driver1/Joint_Driver_5/Controller/Speed/Step Rate and Direction/IC Analog Output REV ==
  SL : Inport
  Controlled Voltage Source : fl_lib/Electrical/Electrical Sources/Controlled Voltage Source
      settings: SourceProductName=Foundation Library
  ERef : fl_lib/Electrical/Electrical Elements/Electrical Reference
      settings: SourceProductName=Foundation Library
  Simulink-PS Converter : nesl_utility/Simulink-PS Converter  PhysicalDomain=network_engine_domain  SubClassName=ps_input  LeftPortType=input  RightPortType=output  PseudoPeriodic=off  Frequencies=[]  NoiseDistribution=none  NoiseParameters=[]  Unit=V  AffineConversion=off  FilteringAndDerivatives=zero  SimscapeFilterOrder=1  InputFilterTimeConstant=.001  UdotUserProvided=0
  V : PMIOPort  Side=Right
  wires:
  SL/1 -> Simulink-PS Converter/1
  connections:
  ERef/LConn1 -- Controlled Voltage Source/RConn2
  V/RConn1 -- Controlled Voltage Source/LConn1
  Simulink-PS Converter/RConn1 -- Controlled Voltage Source/RConn1

== system ROCR6II_URDF_file_915/Driver1/Joint_Driver_5/Controller/Speed/Step Rate and Direction/IC Analog Output Vref ==
  SL : Inport
  Controlled Voltage Source : fl_lib/Electrical/Electrical Sources/Controlled Voltage Source
      settings: SourceProductName=Foundation Library
  ERef : fl_lib/Electrical/Electrical Elements/Electrical Reference
      settings: SourceProductName=Foundation Library
  Simulink-PS Converter : nesl_utility/Simulink-PS Converter  PhysicalDomain=network_engine_domain  SubClassName=ps_input  LeftPortType=input  RightPortType=output  PseudoPeriodic=off  Frequencies=[]  NoiseDistribution=none  NoiseParameters=[]  Unit=V  AffineConversion=off  FilteringAndDerivatives=zero  SimscapeFilterOrder=1  InputFilterTimeConstant=.001  UdotUserProvided=0
  V : PMIOPort  Side=Right
  wires:
  SL/1 -> Simulink-PS Converter/1
  connections:
  Simulink-PS Converter/RConn1 -- Controlled Voltage Source/RConn1
  V/RConn1 -- Controlled Voltage Source/LConn1
  ERef/LConn1 -- Controlled Voltage Source/RConn2

== system ROCR6II_URDF_file_915/Driver1/Joint_Driver_6/Controller/Position/Algorithm and Pulse Generation/IC Analog Output REV ==
  SL : Inport
  Controlled Voltage Source : fl_lib/Electrical/Electrical Sources/Controlled Voltage Source
      settings: SourceProductName=Foundation Library
  ERef : fl_lib/Electrical/Electrical Elements/Electrical Reference
      settings: SourceProductName=Foundation Library
  Simulink-PS Converter : nesl_utility/Simulink-PS Converter  PhysicalDomain=network_engine_domain  SubClassName=ps_input  LeftPortType=input  RightPortType=output  PseudoPeriodic=off  Frequencies=[]  NoiseDistribution=none  NoiseParameters=[]  Unit=V  AffineConversion=off  FilteringAndDerivatives=zero  SimscapeFilterOrder=1  InputFilterTimeConstant=.001  UdotUserProvided=0
  V : PMIOPort  Side=Right
  wires:
  SL/1 -> Simulink-PS Converter/1
  connections:
  ERef/LConn1 -- Controlled Voltage Source/RConn2
  V/RConn1 -- Controlled Voltage Source/LConn1
  Simulink-PS Converter/RConn1 -- Controlled Voltage Source/RConn1

== system ROCR6II_URDF_file_915/Driver1/Joint_Driver_6/Controller/Position/Algorithm and Pulse Generation/IC Analog Output Vref ==
  SL : Inport
  Controlled Voltage Source : fl_lib/Electrical/Electrical Sources/Controlled Voltage Source
      settings: SourceProductName=Foundation Library
  ERef : fl_lib/Electrical/Electrical Elements/Electrical Reference
      settings: SourceProductName=Foundation Library
  Simulink-PS Converter : nesl_utility/Simulink-PS Converter  PhysicalDomain=network_engine_domain  SubClassName=ps_input  LeftPortType=input  RightPortType=output  PseudoPeriodic=off  Frequencies=[]  NoiseDistribution=none  NoiseParameters=[]  Unit=V  AffineConversion=off  FilteringAndDerivatives=zero  SimscapeFilterOrder=1  InputFilterTimeConstant=.001  UdotUserProvided=0
  V : PMIOPort  Side=Right
  wires:
  SL/1 -> Simulink-PS Converter/1
  connections:
  Simulink-PS Converter/RConn1 -- Controlled Voltage Source/RConn1
  V/RConn1 -- Controlled Voltage Source/LConn1
  ERef/LConn1 -- Controlled Voltage Source/RConn2

== system ROCR6II_URDF_file_915/Driver1/Joint_Driver_6/Controller/Position/Algorithm and Pulse Generation/Pulse Generator ==
  Pulse  demand : Inport  SampleTime=1/f
  -1 : Gain  Gain=-1
  Abs : Abs
  Product : Product  InputSameDT=on  SaturateOnIntegerOverflow=on  OutDataTypeStr=Inherit: Same as first input
  Pulse Generator : Subsystem
  Rate Transition : RateTransition  Deterministic=off
  Saturation : Saturate  UpperLimit=1  LowerLimit=-1
  Sign : Signum
  Sum : Sum  Inputs=|+-
  Sum1 : Sum  Inputs=|++
  "Unit Delay, sample time 1/f" : UnitDelay  SampleTime=1/f  HasFrameUpgradeWarning=on
  "[0,1]" : Saturate  UpperLimit=1  LowerLimit=0
  Pulse train : Outport  VectorParamsAs1DForOutWhenUnconnected=off
  Pulse direction : Outport  Port=2  VectorParamsAs1DForOutWhenUnconnected=off
  wires:
  "[0,1]"/1 -> Pulse direction/1
  -1/1 -> Sign/1
  "Unit Delay, sample time 1/f"/1 -> Sum/2, Sum1/2
  Pulse  demand/1 -> Sum/1
  Sum/1 -> -1/1, Saturation/1
  Saturation/1 -> Sum1/1, Abs/1
  Sum1/1 -> "Unit Delay, sample time 1/f"/1
  Sign/1 -> "[0,1]"/1
  Product/1 -> Pulse train/1
  Abs/1 -> Rate Transition/1
  Pulse Generator/1(p) -> Product/2
  Rate Transition/1 -> Product/1

== system ROCR6II_URDF_file_915/Driver1/Joint_Driver_6/Controller/Speed/Step Rate and Direction/IC Analog Output REV ==
  SL : Inport
  Controlled Voltage Source : fl_lib/Electrical/Electrical Sources/Controlled Voltage Source
      settings: SourceProductName=Foundation Library
  ERef : fl_lib/Electrical/Electrical Elements/Electrical Reference
      settings: SourceProductName=Foundation Library
  Simulink-PS Converter : nesl_utility/Simulink-PS Converter  PhysicalDomain=network_engine_domain  SubClassName=ps_input  LeftPortType=input  RightPortType=output  PseudoPeriodic=off  Frequencies=[]  NoiseDistribution=none  NoiseParameters=[]  Unit=V  AffineConversion=off  FilteringAndDerivatives=zero  SimscapeFilterOrder=1  InputFilterTimeConstant=.001  UdotUserProvided=0
  V : PMIOPort  Side=Right
  wires:
  SL/1 -> Simulink-PS Converter/1
  connections:
  Simulink-PS Converter/RConn1 -- Controlled Voltage Source/RConn1
  V/RConn1 -- Controlled Voltage Source/LConn1
  ERef/LConn1 -- Controlled Voltage Source/RConn2

== system ROCR6II_URDF_file_915/Driver1/Joint_Driver_6/Controller/Speed/Step Rate and Direction/IC Analog Output Vref ==
  SL : Inport
  Controlled Voltage Source : fl_lib/Electrical/Electrical Sources/Controlled Voltage Source
      settings: SourceProductName=Foundation Library
  ERef : fl_lib/Electrical/Electrical Elements/Electrical Reference
      settings: SourceProductName=Foundation Library
  Simulink-PS Converter : nesl_utility/Simulink-PS Converter  PhysicalDomain=network_engine_domain  SubClassName=ps_input  LeftPortType=input  RightPortType=output  PseudoPeriodic=off  Frequencies=[]  NoiseDistribution=none  NoiseParameters=[]  Unit=V  AffineConversion=off  FilteringAndDerivatives=zero  SimscapeFilterOrder=1  InputFilterTimeConstant=.001  UdotUserProvided=0
  V : PMIOPort  Side=Right
  wires:
  SL/1 -> Simulink-PS Converter/1
  connections:
  ERef/LConn1 -- Controlled Voltage Source/RConn2
  V/RConn1 -- Controlled Voltage Source/LConn1
  Simulink-PS Converter/RConn1 -- Controlled Voltage Source/RConn1

== system ROCR6II_URDF_file_915/Driver1/Joint_Driver_1/Controller/Position/Algorithm and Pulse Generation/Pulse Generator/Pulse Generator ==
  -1 : Gain  Gain=0.5
  Constant : Constant  SampleTime=1/(2*f)
  Gain : Gain  Gain=-1
  Sum : Sum  Inputs=|++
  "Unit Delay, sample time 1/2*f)" : UnitDelay  InitialCondition=-1  SampleTime=1/(2*f)  HasFrameUpgradeWarning=on
  p : Outport  VectorParamsAs1DForOutWhenUnconnected=off
  wires:
  -1/1 -> p/1
  Sum/1 -> -1/1
  Constant/1 -> Sum/2
  Gain/1 -> "Unit Delay, sample time 1/2*f)"/1
  "Unit Delay, sample time 1/2*f)"/1 -> Sum/1, Gain/1

== system ROCR6II_URDF_file_915/Driver1/Joint_Driver_2/Controller/Position/Algorithm and Pulse Generation/Pulse Generator/Pulse Generator ==
  -1 : Gain  Gain=0.5
  Constant : Constant  SampleTime=1/(2*f)
  Gain : Gain  Gain=-1
  Sum : Sum  Inputs=|++
  "Unit Delay, sample time 1/2*f)" : UnitDelay  InitialCondition=-1  SampleTime=1/(2*f)  HasFrameUpgradeWarning=on
  p : Outport  VectorParamsAs1DForOutWhenUnconnected=off
  wires:
  "Unit Delay, sample time 1/2*f)"/1 -> Gain/1, Sum/1
  Gain/1 -> "Unit Delay, sample time 1/2*f)"/1
  Constant/1 -> Sum/2
  Sum/1 -> -1/1
  -1/1 -> p/1

== system ROCR6II_URDF_file_915/Driver1/Joint_Driver_3/Controller/Position/Algorithm and Pulse Generation/Pulse Generator/Pulse Generator ==
  -1 : Gain  Gain=0.5
  Constant : Constant  SampleTime=1/(2*f)
  Gain : Gain  Gain=-1
  Sum : Sum  Inputs=|++
  "Unit Delay, sample time 1/2*f)" : UnitDelay  InitialCondition=-1  SampleTime=1/(2*f)  HasFrameUpgradeWarning=on
  p : Outport  VectorParamsAs1DForOutWhenUnconnected=off
  wires:
  -1/1 -> p/1
  Sum/1 -> -1/1
  Constant/1 -> Sum/2
  Gain/1 -> "Unit Delay, sample time 1/2*f)"/1
  "Unit Delay, sample time 1/2*f)"/1 -> Sum/1, Gain/1

== system ROCR6II_URDF_file_915/Driver1/Joint_Driver_4/Controller/Position/Algorithm and Pulse Generation/Pulse Generator/Pulse Generator ==
  -1 : Gain  Gain=0.5
  Constant : Constant  SampleTime=1/(2*f)
  Gain : Gain  Gain=-1
  Sum : Sum  Inputs=|++
  "Unit Delay, sample time 1/2*f)" : UnitDelay  InitialCondition=-1  SampleTime=1/(2*f)  HasFrameUpgradeWarning=on
  p : Outport  VectorParamsAs1DForOutWhenUnconnected=off
  wires:
  "Unit Delay, sample time 1/2*f)"/1 -> Gain/1, Sum/1
  Gain/1 -> "Unit Delay, sample time 1/2*f)"/1
  Constant/1 -> Sum/2
  Sum/1 -> -1/1
  -1/1 -> p/1

== system ROCR6II_URDF_file_915/Driver1/Joint_Driver_5/Controller/Position/Algorithm and Pulse Generation/Pulse Generator/Pulse Generator ==
  -1 : Gain  Gain=0.5
  Constant : Constant  SampleTime=1/(2*f)
  Gain : Gain  Gain=-1
  Sum : Sum  Inputs=|++
  "Unit Delay, sample time 1/2*f)" : UnitDelay  InitialCondition=-1  SampleTime=1/(2*f)  HasFrameUpgradeWarning=on
  p : Outport  VectorParamsAs1DForOutWhenUnconnected=off
  wires:
  -1/1 -> p/1
  Sum/1 -> -1/1
  Constant/1 -> Sum/2
  Gain/1 -> "Unit Delay, sample time 1/2*f)"/1
  "Unit Delay, sample time 1/2*f)"/1 -> Sum/1, Gain/1

== system ROCR6II_URDF_file_915/Driver1/Joint_Driver_6/Controller/Position/Algorithm and Pulse Generation/Pulse Generator/Pulse Generator ==
  -1 : Gain  Gain=0.5
  Constant : Constant  SampleTime=1/(2*f)
  Gain : Gain  Gain=-1
  Sum : Sum  Inputs=|++
  "Unit Delay, sample time 1/2*f)" : UnitDelay  InitialCondition=-1  SampleTime=1/(2*f)  HasFrameUpgradeWarning=on
  p : Outport  VectorParamsAs1DForOutWhenUnconnected=off
  wires:
  "Unit Delay, sample time 1/2*f)"/1 -> Gain/1, Sum/1
  Gain/1 -> "Unit Delay, sample time 1/2*f)"/1
  Constant/1 -> Sum/2
  Sum/1 -> -1/1
  -1/1 -> p/1
